simulink model "project_kalman_baseline"  (R2019b)
settings: Solver=FixedStepAuto  StartTime=0.0  StopTime=30  FixedStep=t_sample  RelTol=1e-3
values from neighbouring files (symbols this model uses):
  Ad = sysd.A    [model.m]
  Bd = sysd.B    [model.m]
  Cd = sysd.C    [model.m]
  Ks = Ks'    [model.m]
  Qx = 0.0000001 * eye(4)    [model.m]
  Ry = 0.0000001 * eye(2)    [model.m]
  X0 = [0 0 0 0]'    [baseline_kernel_init.m]    (also in model.m = [0;0;0;0])
  Xm0 = gaussian_noise(X0,100*Pq)    [baseline_kernel_init.m]    (also in model.m = (Ad - Ks * Cd * Ad) * Xm0 + Bd * U(:,k) + Ks*Y(:,k))
undefined symbols (not defined in the file or in its folder): Kd
settings Model: Creator=jania  LastModifiedBy=jania

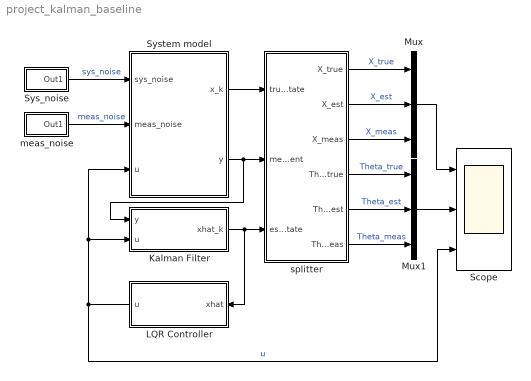
== system project_kalman_baseline ==
  Kalman Filter : Subsystem
  LQR Controller : Subsystem
  Mux : Mux  Inputs=3
  Mux1 : Mux  Inputs=3
  Scope : Scope  NumInputPorts=3
  "Sys_noise " : Subsystem
  System model : Subsystem
  meas_noise : Subsystem
  splitter : Subsystem
  wires:
  Mux1/1 -> Scope/2
  Mux/1 -> Scope/1
  Kalman Filter/1(xhat_k) -> splitter/3(est_state), LQR Controller/1(xhat)
  LQR Controller/1(u) -> System model/3(u), Kalman Filter/2(u), Scope/3  "u"
  System model/2(y) -> splitter/2(measurement), Kalman Filter/1(y)
  "Sys_noise "/1(Out1) -> System model/1(sys_noise)  "sys_noise"
  meas_noise/1(Out1) -> System model/2(meas_noise)  "meas_noise"
  System model/1(x_k) -> splitter/1(true_state)
  splitter/1(X_true) -> Mux/1  "X_true"
  splitter/2(X_est) -> Mux/2  "X_est"
  splitter/3(X_meas) -> Mux/3  "X_meas"
  splitter/4(Theta_true) -> Mux1/1  "Theta_true"
  splitter/5(Theta_est) -> Mux1/2  "Theta_est"
  splitter/6(Theta_meas) -> Mux1/3  "Theta_meas"

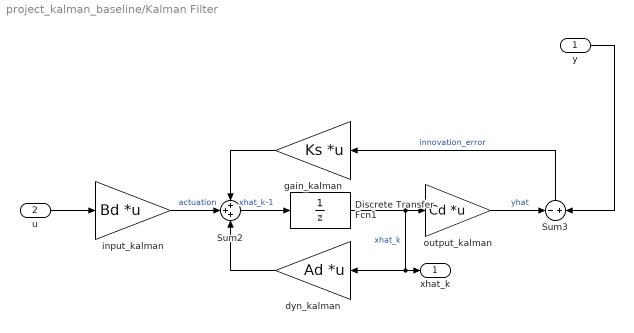
== system project_kalman_baseline/Kalman Filter ==
  y : Inport
  u : Inport  Port=2
  Discrete Transfer Fcn1 : DiscreteTransferFcn  Denominator=[1 0]  InitialStates=Xm0
  Sum2 : Sum  Inputs=+++
  Sum3 : Sum  Inputs=-|+
  dyn_kalman : Gain  Gain=Ad  Multiplication=Matrix(K*u)
  gain_kalman : Gain  Gain=Ks  Multiplication=Matrix(K*u)
  input_kalman : Gain  Gain=Bd  Multiplication=Matrix(K*u)
  output_kalman : Gain  Gain=Cd  Multiplication=Matrix(K*u)
  xhat_k : Outport
  wires:
  input_kalman/1 -> Sum2/2  "actuation"
  dyn_kalman/1 -> Sum2/3
  Sum2/1 -> Discrete Transfer Fcn1/1  "xhat_k-1"
  Discrete Transfer Fcn1/1 -> dyn_kalman/1, xhat_k/1, output_kalman/1  "xhat_k"
  y/1 -> Sum3/2
  Sum3/1 -> gain_kalman/1  "innovation_error"
  output_kalman/1 -> Sum3/1  "yhat"
  gain_kalman/1 -> Sum2/1
  u/1 -> input_kalman/1

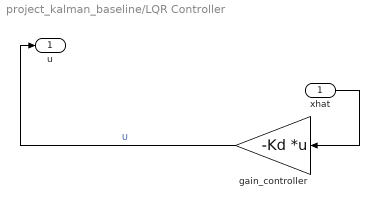
== system project_kalman_baseline/LQR Controller ==
  xhat : Inport
  "gain_controller " : Gain  Gain=-Kd  Multiplication=Matrix(K*u)
  u : Outport
  wires:
  "gain_controller "/1 -> u/1  "U"
  xhat/1 -> "gain_controller "/1

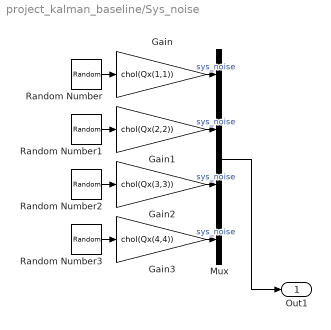
== system project_kalman_baseline/Sys_noise  ==
  Gain : Gain  Gain=chol(Qx(1,1))
  Gain1 : Gain  Gain=chol(Qx(2,2))
  Gain2 : Gain  Gain=chol(Qx(3,3))
  Gain3 : Gain  Gain=chol(Qx(4,4))
  Mux : Mux
  Random Number{,1..3} (4 alike) : RandomNumber
  Out1 : Outport
  wires:
  Gain2/1 -> Mux/3  "sys_noise"
  Random Number3/1 -> Gain3/1
  Gain1/1 -> Mux/2  "sys_noise"
  Gain3/1 -> Mux/4  "sys_noise"
  Random Number/1 -> Gain/1
  Mux/1 -> Out1/1
  Gain/1 -> Mux/1  "sys_noise"
  Random Number1/1 -> Gain1/1
  Random Number2/1 -> Gain2/1

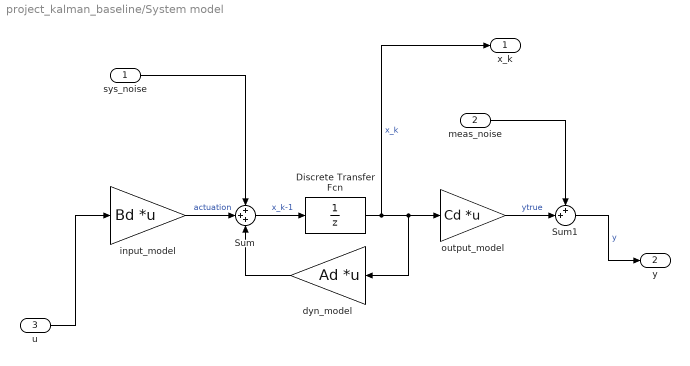
== system project_kalman_baseline/System model ==
  sys_noise : Inport
  meas_noise : Inport  Port=2
  u : Inport  Port=3
  Discrete Transfer Fcn : DiscreteTransferFcn  Denominator=[1 0]  InitialStates=X0
  Sum : Sum  Inputs=+++
  Sum1 : Sum  Inputs=++|
  dyn_model : Gain  Gain=Ad  Multiplication=Matrix(K*u)
  input_model : Gain  Gain=Bd  Multiplication=Matrix(K*u)
  output_model : Gain  Gain=Cd  Multiplication=Matrix(K*u)
  x_k : Outport
  y : Outport  Port=2
  wires:
  Discrete Transfer Fcn/1 -> x_k/1, output_model/1, dyn_model/1  "x_k"
  Sum/1 -> Discrete Transfer Fcn/1  "x_k-1"
  meas_noise/1 -> Sum1/1
  input_model/1 -> Sum/2  "actuation"
  sys_noise/1 -> Sum/1
  dyn_model/1 -> Sum/3
  output_model/1 -> Sum1/2  "ytrue"
  u/1 -> input_model/1
  Sum1/1 -> y/1  "y"

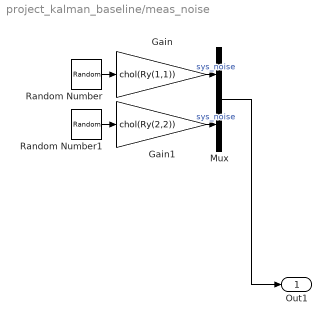
== system project_kalman_baseline/meas_noise ==
  Gain : Gain  Gain=chol(Ry(1,1))
  Gain1 : Gain  Gain=chol(Ry(2,2))
  Mux : Mux  Inputs=2
  Random Number : RandomNumber
  Random Number1 : RandomNumber
  Out1 : Outport
  wires:
  Gain1/1 -> Mux/2  "sys_noise"
  Random Number/1 -> Gain/1
  Mux/1 -> Out1/1
  Gain/1 -> Mux/1  "sys_noise"
  Random Number1/1 -> Gain1/1

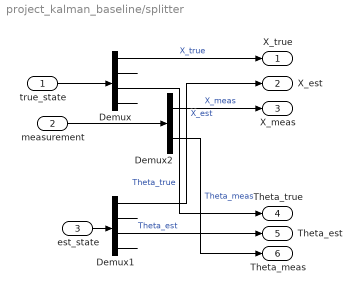
== system project_kalman_baseline/splitter ==
  true_state : Inport
  measurement : Inport  Port=2
  est_state : Inport  Port=3
  Demux : Demux
  Demux1 : Demux
  Demux2 : Demux  Outputs=2
  X_true : Outport
  X_est : Outport  Port=2
  X_meas : Outport  Port=3
  Theta_true : Outport  Port=4
  Theta_est : Outport  Port=5
  Theta_meas : Outport  Port=6
  wires:
  Demux2/2 -> Theta_meas/1  "Theta_meas"
  Demux/1 -> X_true/1  "X_true"
  Demux1/1 -> X_est/1  "X_est"
  Demux/4 -> ?
  measurement/1 -> Demux2/1
  Demux/2 -> ?
  Demux1/3 -> Theta_est/1  "Theta_est"
  est_state/1 -> Demux1/1
  Demux1/4 -> ?
  Demux/3 -> Theta_true/1  "Theta_true"
  Demux1/2 -> ?
  true_state/1 -> Demux/1
  Demux2/1 -> X_meas/1  "X_meas"
